simulink library "APST_Lib"  (R2016a)
settings: Solver=ode45  StartTime=0.0  StopTime=10.0  RelTol=1e-3
undefined symbols (not defined in the file or in its folder): ACM, COMP_MAP, rev_comms_sink
libraries: APST_Lib x97
(part 4 of 6)

== system APST_Lib/Thermal Components ==
  "ACM Shaft " : Subsystem  mask(Shaft){N_init=45000, Comp_r1=.05, Comp_r2=.15, m_comp=5, Turb_r1=.15, Turb_r2=.1, m_turb=5, PComp_r1=0.05, PComp_r2=0.025, m_pcomp=5, Shft_r=.05, m_shft=10, J_comp=0.034904, J_turb=0.041645, J_pcomp=0.0041518, J_shaft=0.0125}
      mask prompts: N_init "Initial Rotational Speed [RPM]"; Comp_r1 "Entrance Tip Radius [m]"; Comp_r2 "Exit Tip Radius [m]"; m_comp "Mass [kg]"; Turb_r1 "Entrance Tip Radius [m]"; Turb_r2 "Exit Tip Radius [m]"; m_turb "Mass [kg]"; PComp_r1 "Entrance Tip Radius [m]"; PComp_r2 "Exit Tip Radius [m]"; m_pcomp "Mass [kg]"; Shft_r "Radius [m]"; m_shft "Mass [kg]"; J_comp "Compressor"; J_turb "Expansion Turbine"; J_pcomp "Power Compressor"; J_shaft "ACM Shaft"
      mask init:
      | load Fluids
      | eval(['Air = Fluid.Air;']);
      | 
      | J_comp = (3/10) * m_comp * (Comp_r2^5 - Comp_r1^5) / (Comp_r2^3 - Comp_r1^3);
      | set_param(gcb,'J_comp',num2str(J_comp));
      | 
      | J_turb = (3/10) * m_comp * (Turb_r1^5 - Turb_r2^5) / (Turb_r1^3 - Turb_r2^3);
      | set_param(gcb,'J_turb',num2str(J_turb));
      | 
      | J_pcomp = (3/10) * m_comp * (PComp_r1^5 - PComp_r2^5) / (PComp_r1^3 - PComp_r2^3);
      | set_param(gcb,'J_pcomp',num2str(J_pcomp));
      | 
      | J_shaft = (1/2) * m_shft * Shft_r^2;
      | set_param(gcb,'J_shaft',num2str(J_shaft));
  Air Volume : Subsystem  mask(Air volume){fld=Air, T_init=22, M_init=262.8177, P_init=105, Tamb_init=22, H=0, D=3, L=30, V=212.0575, A_sa=282.7433, Pamb=101, E_fluid=101*1e3}
      mask prompts: fld "Fluid Type"; T_init "Initial Air Temperature [°C]"; M_init "Initial Fluid Mass [kg]"; P_init "Air Pressure [kPa]"; Tamb_init "Initial Ambient Temperature [°C]"; H "Heat Transfer Coefficient with Ambient [W/m²K]"; D "Air Volume Diameter [m]"; L "Air Volume Length [m]"; V "Air Volume [m³]"; A_sa "Air Volume Surface Area [m²]"; Pamb "Ambient Pressure [kPa]"; E_fluid "Bulk Modulus"
      mask help: Tracks the time rate of change for fluid mass and temperature.
      mask init:
      | load('Fluids.mat');
      | Fluid = eval(['Fluid.',fld]);
      | 
      | % calculate the volume -- assuming a cylinder
      | V = L*pi*D^2/4;    
      | set_param(gcb,'V',num2str(V));
      | 
      | % calculate the surface area -- assuming a cylinder
      | SA = L * pi * D ;
      | set_param(gcb,'A_sa',num2str(SA));
      | 
      | % Note: Assumes a fixed initial pressure to calculate density
      | P_for_rho = 105;
      | Rho = qminterp2(Fluid.T, Fluid.P, Fluid.Rho_pt, T_init, P_for_rho);
      | 
      | % set the mass of air in the air volume
      | set_param(gcb,'M_init',num2str(Rho*V));
      settings: OpenFcn=|
      | load('Fluids.mat');
      | Set_Fluid_Popup_Names( Fluid )
      mask TypeOptions fld: Fuel | Water | Air | PG50
      mask DialogControl NomValuesGroupVar Prompt: Component Sizing - Nominal Values
      mask Display:
      | image(imread('cabin.png'))
      | 
      | text(0.5,0.9,['{\bf Air Volume}'],'TexMode','on','horizontalAlignment', 'center')
      | text(0.5,0.1,['{(P)}'],'TexMode','on','horizontalAlignment', 'center')
      | 
      | port_label('input',1,'Flow In')
      | port_label('input',2,'Amb. Temp. [°C]')
      | port_label('input',3,'Q internal [kW]')
      | port_label('output',1,'Flow Out')
      | % port_label('output',2,'Fluid Mass [kg]')
  Cold Plate : Subsystem  mask(Cold Plate){fld=Fuel, P_init=101, Tw_init=22, T_init=22, f=0.05, KL=0, PAF=1, M_wall=0.77632, Cp_wall=.9, H1=2000, D=0.007, L=0.75, t=0.0015, E=2.4e6, v=0.4, dH=0, e_rough=0.0015*1e-3}
      mask prompts: fld "Fluid Type"; P_init "Initial Outlet Pressure [kPa]"; Tw_init "Initial Wall Temperature [°C]"; T_init "Initial Outlet Temperature [°C]"; f "Friction Factor [-]"; KL "Minor Losses [-]"; PAF "HTC Parameter Adjustment Factor [-]"; M_wall "Wall Mass [kg]"; Cp_wall "Wall Specific Heat [kJ/kg*K]"; H1 "Heat Transfer Coeff. [W/m²K]"; D "Internal Diameter [m]"; L "Tube Length [m]"; t "Tube Wall Thickness [m]"; E "Tube Modulus of Elasticity [kPa]"; v "Tube Poisson Ratio [-]"; dH "Height between Inlet and Outlet [m]"; e_rough "Surface Roughness [m] (0.0015mm for copper, 0.01mm for rubber, 0mm for plastic)"
      mask help: Tracks the time rate of change of the pressure, wall temperature, and fluid exit temperature.
      mask init:
      | load('Fluids.mat');
      | Fluid = eval(['Fluid.',fld]);
      | 
      | load('Moody.mat');
      settings: OpenFcn=|
      | load('Fluids.mat');
      | Set_Fluid_Popup_Names( Fluid )
      mask TypeOptions fld: Fuel | Water | Air | PG50
      mask DialogControl Container13 Prompt: Component Sizing - Nominal Values
      mask Display:
      | image(imread('ColdPlate.jpg'))
      | 
      | text(0.5,0.95,['{\bf ',fld,' Cold Plate}'],'TexMode','on','horizontalAlignment', 'center')
      | text(0.5,0.08,['{-----(P)}'],'TexMode','on','horizontalAlignment', 'center')
      | 
      | port_label('input',1,'Flow In')
      | port_label('input',2,'Heat Load [kW]')
      | port_label('output',1,'Flow Out')
  Compressor : Subsystem  mask(Centrifugal Compressor){COMP=ACM.MAP.PwrComp, init_mdot=0}
      mask prompts: COMP "Workspace Variable:"; init_mdot "Initial Mass Flow Rate"
      mask help:
      | Input #1: Flow conditions at compressor inlet [kPa, °C]
      | Input #2: RPM of the compressor shaft [RPM]
      |
      | Output #1: Flow conditions at compressor outlet [kg/s, kPa, °C]
      | Output #2: Power consumed by the compressor [W]
      mask Display:
      | image(imread('compressor.png'))
      | 
      | text(0.5,0.95,['{\bf Compressor}'],'TexMode','on','horizontalAlignment', 'center')
      | text(0.5,0.08,['{----}'],'TexMode','on','horizontalAlignment', 'center')
      | 
      | port_label('input',1,'Flow In')
      | port_label('input',2,'RPM')
      | 
      | port_label('output',1,'Flow Out #')
      | port_label('output',2,'Power [W]')
  Fan : Subsystem  mask(Liquid Pump){P_init=145, T_init=22, D=13*1e-3, L=0.1, rho=1000, cp=4, E=0, Omega_max=3000, DP_max=20, mdot_max=0.5, alpha=0.001}
      mask prompts: P_init "Intial Outlet Pressure [kPa]"; T_init "Intial Outlet Temperature [°C]"; D "Pipe Internal Diameter [m]"; L "Pipe Length [m]"; rho "Air Density [kg/m^3]"; cp "Air Specific Heat [kJ/kgK]"; E "Air Modulus of Elasticity [N/m^2]"; Omega_max "Maximum Shaft Speed [RPM]"; DP_max "Maximum Pressure Difference [kPa]"; mdot_max "Maximum Mass Flow Rate [kg/s]"; alpha "Heat Generation Coefficient [kW/RPM]"
      mask help: Tracks the time rate of change of fluid temperature, mass flow rate, and power consumption.
      mask init:
      | load('Fluids.mat');
      | Fluid = eval(['Fluid.Air']);
      settings: OpenFcn=|
      | load('Fluids.mat');
      | Set_Fluid_Popup_Names( Fluid )
      mask DialogControl Container15 Prompt: Component Sizing - Nominal Values
      mask Display:
      | % image(imread('centpump.jpg'))
      | 
      | text(0.5,0.95,['{\bf Fan}'],'TexMode','on','horizontalAlignment', 'center')
      | text(0.5,0.1,['{-----(P)}'],'TexMode','on','horizontalAlignment', 'center')
      | 
      | port_label('input',1,'Flow In')
      | port_label('input',2,'Power')
      | port_label('input',3,'Shaft Speed [RPM]')
      | port_label('output',1,'Flow Out')
  Flow Split_Junction : Subsystem  mask(Split/Junction){fld=Fuel, Num_Out=1, Num_In=1, P_init=110, T_init=22, D=0.013, L=0.1, t=0.0015, E=2.4e6, v=0.4}
      mask prompts: fld "Fluid Type"; Num_Out "Number of Outlet Flows"; Num_In "Number of Inlet Flows"; P_init "Initial Pressure [kPa]"; T_init "Initial Temperature [°C]"; D "Diameter [m]"; L "Length [m]"; t "Tube Wall Thickness [m]"; E "Tube Modulus of Elasticity [kPa]"; v "Tube Poisson Ratio [-]"
      mask help: Splits and junctions flows using dynamic relationships. Note that the library link of the block is disabled when it is imported into a model.
      mask init:
      | h      = get_param(gcb,'handle');   % Get block handle
      | blk    = gcb;
      | hblock = get(h);     % Parse out handles structure
      | 
      | load('Fluids.mat');
      | Fluid = eval(['Fluid.',fld]);
      | 
      | % delete any previous inports and bus selectors
      | for i = str2num(hblock.Num_In)+1:hblock.Ports(1)
      |     delete_block([blk,'/In',num2str(i)])
      |     delete_block([blk,'/gb',num2str(i)])
      |     delete_block([blk,'/gm',num2str(i)])
      |     delete_block([blk,'/gt',num2str(i)])
      |     delete_block([blk,'/gp',num2str(i)])
      |     delete_block([blk,'/Sink',num2str(i)])
      |     delete_block([blk,'/pout',num2str(i)])
      |     delete_block([blk,'/min',num2str(i)])
      |     delete_block([blk,'/tin',num2str(i)])
      |     
      |     delete_unconnected_lines(blk)
      | end
      | 
      | % delete any previous inports and bus selectors
      | for i = str2num(hblock.Num_Out)+1:hblock.Ports(2)
      |     delete_block([blk,'/Out',num2str(i)])
      |     delete_block([blk,'/m',num2str(i)])
      |     delete_block([blk,'/t',num2str(i)])
      |     delete_block([blk,'/p',num2str(i)])
      |     delete_block([blk,'/b',num2str(i)])
      |     delete_block([blk,'/Source',num2str(i)])
      |     delete_block([blk,'/g',num2str(i)])
      |     delete_block([blk,'/mout',num2str(i)])
      |     %delete_block([blk,'/tout',num2str(i)])
      |     
      |     delete_unconnected_lines(blk)
      | end
      | 
      | set_param([blk,'/Mux_In_1'],'Inputs',hblock.Num_In)
      | set_param([blk,'/Mux_In_2'],'Inputs',hblock.Num_Out)
      | set_param([blk,'/Mux_In_3'],'Inputs',hblock.Num_In)
      | %set_param([blk,'/Mux_Out_1'],'Outputs',hblock.Num_Out)
      | 
      | % generate inports, bus selectors, and route lines to each vector concat
      | for i = hblock.Ports(1)+1:str2num(hblock.Num_In)
      |     
      |     % add blocks
      |     add_block('simulink/Ports & Subsystems/In1',   [blk,'/In',num2str(i)],    'Position',[120 i*80-25+20 150 i*80-12+20]);         % adding inport
      |     add_block([blk,'/gb1'],                        [blk,'/gb',num2str(i)],   'Position',[200 i*80-20+20-18 205 i*80-2+20+2]);         % adding inport
      |     add_block('simulink/Signal Routing/Goto',      [blk,'/gm',num2str(i)],    'Position',[260 i*80-17 340 i*80-3]);         % adding inport
      |     add_block('simulink/Signal Routing/Goto',      [blk,'/gt',num2str(i)],    'Position',[260 i*80+3 340 i*80+17]);         % adding inport
      |     add_block('simulink/Sinks/Terminator',          [blk,'/gp',num2str(i)],    'Position',[260 i*80+23 280 i*80+37]);         % adding inport
      |     add_block('APST_Lib/Support Components/Sink',[blk,'/Sink',num2str(i)],'Position',[745 i*80-14 810 i*80+14]);         % adding inport
      |     add_block('simulink/Signal Routing/From',      [blk,'/pout',num2str(i)],    'Position',[625 i*80-14 705 i*80+14]);         % adding inport
      |     add_block('simulink/Signal Routing/From',       [blk,'/min',num2str(i)],     'Position',[935 -258+i*20 1015 -242+i*20]);         % adding inport
      |     add_block('simulink/Signal Routing/From',       [blk,'/tin',num2str(i)],     'Position',[935 1+i*20 1015 19+i*20]);         % adding inport
      |     
      |     % set goto and from tags
      |     set_param([blk,'/gm',num2str(i)],'GotoTag',char(horzcat('M_in',num2str(i))))
      |     set_param([blk,'/gt',num2str(i)],'GotoTag',char(horzcat('T_in',num2str(i))))
      |     %set_param([blk,'/gp',num2str(i)],'GotoTag',char(horzcat('P_in',num2str(i))))
      |     set_param([blk,'/pout',num2str(i)],'GotoTag',char('P'))
      |     set_param([blk,'/min',num2str(i)],'GotoTag',char(horzcat('M_in',num2str(i))))
      |     set_param([blk,'/tin',num2str(i)],'GotoTag',char(horzcat('T_in',num2str(i))))
      |     
      |     % set goto and from background colors
      |     set_param([blk,'/gm',num2str(i)],'BackgroundColor','yellow')
      |     set_param([blk,'/gt',num2str(i)],'BackgroundColor','yellow')
      |     %set_param([blk,'/gp',num2str(i)],'BackgroundColor','yellow')
      |     set_param([blk,'/min',num2str(i)],'BackgroundColor','yellow')
      |     set_param([blk,'/tin',num2str(i)],'BackgroundColor','yellow')
      |     set_param([blk,'/pout',num2str(i)],'BackgroundColor','cyan')
      |     
      |     % add lines
      |     add_line(blk,['In',num2str(i),'/1'], ['gb',num2str(i),'/1'],'AutoRouting','on')
      |     add_line(blk,['gb',num2str(i),'/1'],  ['gm',num2str(i),'/1'],'AutoRouting','on')
      |     add_line(blk,['gb',num2str(i),'/2'],  ['gt',num2str(i),'/1'],'AutoRouting','on')
      |     add_line(blk,['gb',num2str(i),'/3'],  ['gp',num2str(i),'/1'],'AutoRouting','on')
      |     add_line(blk,['pout',num2str(i),'/1'],  ['Sink',num2str(i),'/1'],'AutoRouting','on')
      |     add_line(blk,['min',num2str(i),'/1'],  ['Mux_In_1/',num2str(i)],'AutoRouting','on')
      |     add_line(blk,['tin',num2str(i),'/1'],  ['Mux_In_3/',num2str(i)],'AutoRouting','on')
      |     
      | end
      | 
      | % generate inports, bus selectors, and route lines to each vector concat
      | for i = hblock.Ports(2)+1:str2num(hblock.Num_Out)
      |     
      |     % add blocks
      |     add_block('simulink/Ports & Subsystems/Out1',   [blk,'/Out',num2str(i)],   'Position',[30 i*80-25+20 60 i*80-12+20]);         % adding inport
      |     add_block('simulink/Signal Routing/From',       [blk,'/m',num2str(i)],     'Position',[-150 i*80-20 -70 i*80-2]);         % adding inport
      |     add_block('simulink/Signal Routing/From',       [blk,'/t',num2str(i)],     'Position',[-150 i*80-20+20 -70 i*80-2+20]);         % adding inport
      |     add_block('simulink/Signal Routing/From',       [blk,'/p',num2str(i)],     'Position',[-150 i*80-20+40 -70 i*80-2+40]);         % adding inport
      |     add_block('simulink/Signal Routing/Bus Creator',[blk,'/b',num2str(i)],     'Position',[5 i*80-20+20-18 10 i*80-2+20+2]);         % adding inport
      |     add_block('APST_Lib/Support Components/Source',[blk,'/Source',num2str(i)],'Position',[395 i*80-14 460 i*80+14]);         % adding inport
      |     add_block('simulink/Signal Routing/Goto',       [blk,'/g',num2str(i)],     'Position',[505 i*80-9 585 i*80+9]);         % adding inport
      |     add_block('simulink/Signal Routing/From',       [blk,'/mout',num2str(i)],  'Position',[935 -129+i*20 1015 -111+i*20]);         % adding inport
      |     %add_block('simulink/Signal Routing/Goto',      [blk,'/tout',num2str(i)],   'Position',[1455 -259+i*20 1535 -241+i*20]);         % adding inport
      |     
      |     % set goto and from tags
      |     set_param([blk,'/m',num2str(i)],'GotoTag',char(horzcat('M_out',num2str(i))))
      |     %set_param([blk,'/t',num2str(i)],'GotoTag',char(horzcat('T_out',num2str(i))))
      |     set_param([blk,'/t',num2str(i)],'GotoTag',char('T'))
      |     set_param([blk,'/p',num2str(i)],'GotoTag',char('P'))
      |     set_param([blk,'/g',num2str(i)],'GotoTag',char(horzcat('M_out',num2str(i))))
      |     set_param([blk,'/mout',num2str(i)],'GotoTag',char(horzcat('M_out',num2str(i))))
      |     %set_param([blk,'/tout',num2str(i)],'GotoTag',char(horzcat('T_out',num2str(i))))
      |     set_param([blk,'/b',num2str(i)],'Inputs','3')
      |     
      |     % set goto and from background colors
      |     set_param([blk,'/t',num2str(i)],'BackgroundColor','cyan')
      |     set_param([blk,'/m',num2str(i)],'BackgroundColor','cyan')
      |     set_param([blk,'/p',num2str(i)],'BackgroundColor','cyan')
      |     set_param([blk,'/g',num2str(i)],'BackgroundColor','cyan')
      |     set_param([blk,'/mout',num2str(i)],'BackgroundColor','cyan')
      |     %set_param([blk,'/tout',num2str(i)],'BackgroundColor','cyan')
      |     
      |     % add lines
      |     add_line(blk,['m',num2str(i),'/1'],['b',num2str(i),'/1'],'AutoRouting','on')
      |     p = get_param([blk,'/m',num2str(i)],'PortHandles');
      |     l = get_param(p.Outport,'Line');
      |     set_param(l,'Name','mdot_kgps')
      |     
      |     add_line(blk,['t',num2str(i),'/1'],['b',num2str(i),'/2'],'AutoRouting','on')
      |     p = get_param([blk,'/t',num2str(i)],'PortHandles');
      |     l = get_param(p.Outport,'Line');
      |     set_param(l,'Name','T_C')
      |     
      |     add_line(blk,['p',num2str(i),'/1'],['b',num2str(i),'/3'],'AutoRouting','on')
      |     p = get_param([blk,'/p',num2str(i)],'PortHandles');
      |     l = get_param(p.Outport,'Line');
      |     set_param(l,'Name','P_kPa')
      |     
      |     add_line(blk,['b',num2str(i),'/1'],['Out',num2str(i),'/1'],'AutoRouting','on')
      |     add_line(blk,['Source',num2str(i),'/1'],['g',num2str(i),'/1'],'AutoRouting','on')
      |     add_line(blk,['mout',num2str(i),'/1'],  ['Mux_In_2/',num2str(i)],'AutoRouting','on')
      |     %add_line(blk,['Mux_Out_1/',num2str(i)], ['tout',num2str(i),'/1'],'AutoRouting','on')
      | end
      | 
      | try
      |     set_param([blk,'/Selector1'],'InputPortWidth',num2str(hblock.Num_In))
      |     set_param([blk,'/Selector2'],'InputPortWidth',num2str(hblock.Num_In))
      |     
      |     selector_str = '[1 ';
      |     for i = 2:str2num(hblock.Num_In)
      |         selector_str = [selector_str,num2str(i),' '];
      |     end
      |     selector_str = [selector_str,']'];
      |     set_param([blk,'/Selector1'],'IndexParamArray',{selector_str})%num2cell(1:hblock.Num_In))
      |     set_param([blk,'/Selector2'],'IndexParamArray',{selector_str})%num2cell(1:hblock.Num_In))
      | catch
      |     selector_str = '[1 ';
      |     for i = 2:str2num(hblock.Num_In)
      |         selector_str = [selector_str,num2str(i),' '];
      |     end
      |     selector_str = [selector_str,']'];
      |     set_param([blk,'/Selector1'],'IndexParamArray',{selector_str})%num2cell(1:hblock.Num_In))
      |     set_param([blk,'/Selector2'],'IndexParamArray',{selector_str})%num2cell(1:hblock.Num_In))
      |     
      |     set_param([blk,'/Selector1'],'InputPortWidth',num2str(hblock.Num_In))
      |     set_param([blk,'/Selector2'],'InputPortWidth',num2str(hblock.Num_In))
      | end 
      |     
      |     clear h blk hblock
      settings: CopyFcn=|
      | h      = get_param(gcb,'handle');   % Get block handle
      | blk    = gcb;
      | 
      | set_param(blk, 'LinkStatus', 'inactive')
      settings: OpenFcn=|
      | load('Fluids.mat');
      | Set_Fluid_Popup_Names( Fluid )
      mask TypeOptions fld: Fuel | Water | Air | PG50
      mask DialogControl Container15 Prompt: Component Sizing - Nominal Values
      mask Display:
      | image(imread('Split.jpg'));
      | 
      | text(0.5,0.95,['{\bf',fld,' Split/Junction}'],'TexMode','on','horizontalAlignment', 'center')
      | text(0.5,0.08,['{(P)}'],'TexMode','on','horizontalAlignment', 'center')
      | 
      | h      = get_param(gcb,'handle');   % Get block handle
      | blk    = gcb;
      | hblock = get(h);     % Parse out handles structure
      | for i = 1:str2num(hblock.Num_In)
      |     port_label('input',i,horzcat('Flow In #',num2str(i)))
      | end
      | for i = 1:str2num(hblock.Num_Out)
      |     port_label('output',i,horzcat('Flow Out #',num2str(i)))
      | end
  Flow Split_Junction1 : Subsystem  mask(Split/Junction){fld=Fuel, Num_Out=2, Num_In=1, P_init=110, T_init=22, D=0.013, L=0.1, t=0.0015, E=2.4e6, v=0.4}
      mask prompts: fld "Fluid Type"; Num_Out "Number of Outlet Flows"; Num_In "Number of Inlet Flows"; P_init "Initial Pressure [kPa]"; T_init "Initial Temperature [°C]"; D "Diameter [m]"; L "Length [m]"; t "Tube Wall Thickness [m]"; E "Tube Modulus of Elasticity [kPa]"; v "Tube Poisson Ratio [-]"
      mask help: Splits and junctions flows using dynamic relationships. Note that the library link of the block is disabled when it is imported into a model.
      mask init:
      | h      = get_param(gcb,'handle');   % Get block handle
      | blk    = gcb;
      | hblock = get(h);     % Parse out handles structure
      | 
      | load('Fluids.mat');
      | Fluid = eval(['Fluid.',fld]);
      | 
      |     
      |     clear h blk hblock
      settings: CopyFcn=|
      | h      = get_param(gcb,'handle');   % Get block handle
      | blk    = gcb;
      | 
      | set_param(blk, 'LinkStatus', 'inactive')
      settings: OpenFcn=|
      | load('Fluids.mat');
      | Set_Fluid_Popup_Names( Fluid )
      mask TypeOptions fld: Fuel | Water | Air | PG50
      mask DialogControl Container15 Prompt: Component Sizing - Nominal Values
      mask Display:
      | image(imread('valve.png'));
      | 
      | text(0.5,0.95,['{\bf',fld,' Valve}'],'TexMode','on','horizontalAlignment', 'center')
      | text(0.5,0.08,['{----}'],'TexMode','on','horizontalAlignment', 'center')
      | 
      | h      = get_param(gcb,'handle');   % Get block handle
      | blk    = gcb;
      | hblock = get(h);     % Parse out handles structure
      | for i = 1:str2num(hblock.Num_In)
      |     port_label('input',i,horzcat('Flow In #',num2str(i)))
      | end
      | port_label('input',2,'Input [0-1]')
      | for i = 1:str2num(hblock.Num_Out)
      |     port_label('output',i,horzcat('Flow Out #',num2str(i)))
      | end
  Fluid Tank : Subsystem  mask(Fluid Tank){fld=Fuel, T_init=22, h_init=0.2, M_init=500, P_init=105, Tamb_init=22, H=0, D=0.08, V=3, A_sa=0, Pamb=101}
      mask prompts: fld "Fluid Type"; T_init "Initial Fluid Temperature [°C]"; h_init "Initial Fluid Height [m]"; M_init "Initial Fluid Mass [kg]"; P_init "Tank Pressure [kPa]"; Tamb_init "Initial Ambient Temperature [°C]"; H "Heat Transfer Coefficient with Ambient [W/m²K]"; D "Tank Diameter [m]"; V "Tank Volume [m³]"; A_sa "Tank Surface Area [m²]"; Pamb "Ambient Pressure [kPa]"
      mask help: Tracks the time rate of change for fluid mass and temperature.
      mask init:
      | load('Fluids.mat');
      | Fluid = eval(['Fluid.',fld]);
      | 
      | % Note: Assumes a fixed initial pressure to calculate density
      | P_for_rho = 105;
      | Rho = qminterp2(Fluid.T, Fluid.P, Fluid.Rho_pt, T_init, P_for_rho);
      | 
      | % M_init = h_init*Rho*pi*D^2/4;
      | M_max = Rho*V;
      | if M_max < M_init
      |     set_param(gcb,'M_init',num2str(M_max));
      |     msgbox('Fuel tank volume is too small for initial mass. Setting initial mass to maximum.')
      | end
      | 
      | % P_init = Rho*9.81*h_init/1000 + Pamb;
      | % set_param(gcb,'P_init',num2str(P_init));
      settings: OpenFcn=|
      | load('Fluids.mat');
      | Set_Fluid_Popup_Names( Fluid )
      mask TypeOptions fld: Fuel | Water | Air | PG50
      mask DialogControl NomValuesGroupVar Prompt: Component Sizing - Nominal Values
      mask Display:
      | image(imread('fueltank.jpg'))
      | 
      | text(0.5,0.9,['{\bf ',fld,' Tank}'],'TexMode','on','horizontalAlignment', 'center')
      | text(0.5,0.1,['{(P)}'],'TexMode','on','horizontalAlignment', 'center')
      | 
      | port_label('input',1,'Flow In')
      | port_label('input',2,'Amb. Temp. [°C]')
      | port_label('input',3,'Q internal [kW]')
      | port_label('output',1,'Flow Out')
      | port_label('output',2,'Fluid Mass [kg]')
  Heat Exchanger : Subsystem  mask(Heat Exchanger){Tw_init=22, fld1=Air, P1_init=95, T1_init=22, f1=0.05, KL1=0, fld2=Air, P2_init=120, T2_init=10, f2=0.05, KL2=0, M_wall=0.1, Cp_wall=0.9, Pass1=5, H1=2000, b1=1*1e-3, W1=87*1e-3, L1=0.193, dH1=0, e1=0.0015*1e-3, Nu_lam1=5.6153, Pass2=5, H2=2000, b2=1*1e-2, W2=87*1e-2, L2=0.193, dH2=0, e2=0.0015*1e-3, Nu_lam2=5.6153}
      mask prompts: Tw_init "Initial Wall Temperature [°C]"; fld1 "Fluid Type 1"; P1_init "Initial Outlet 1 Pressure [kPa]"; T1_init "Initial Outlet 1 Temperature [°C]"; f1 "Friction Factor [-]"; KL1 "Minor Losses [-]"; fld2 "Fluid Type 2"; P2_init "Initial Outlet 2 Pressure [kPa]"; T2_init "Initial Outlet 2 Temperature [°C]"; f2 "Friction Factor [-]"; KL2 "Minor Losses [-]"; M_wall "Single Wall Mass [kg]"; Cp_wall "Wall Specific Heat [kJ/kg*K]"; Pass1 "Number of Passes"; H1 "Heat transfer coeff. [W/m²K]"; b1 "Plate Spacing [m]"; W1 "Plate Width [m]"; L1 "Plate Length [m]"; dH1 "Height between Inlet and Outlet [m]"; e1 "Surface Roughness [m] (0.0015mm for copper, 0.01mm for rubber, 0mm for plastic)"; Nu_lam1 "Laminar Nu"; Pass2 "Number of Passes"; H2 "Heat transfer coeff. [W/m²K]"; b2 "Plate Spacing [m]"; W2 "Plate Width [m]"; L2 "Plate Length [m]"; dH2 "Height between Inlet and Outlet [m]"; e2 "Surface Roughness [m] (0.0015mm for copper, 0.01mm for rubber, 0mm for plastic)"; Nu_lam2 "Laminar Nu"
      mask help: Tracks the time rate of change of the pressure, wall temperature, and exit flow temperatures.
      mask init:
      | load('Fluids.mat');
      | Fluid1 = eval(['Fluid.',fld1]);
      | Fluid2 = eval(['Fluid.',fld2]);
      | 
      | load('Moody.mat');
      | 
      | load('Laminar_Props.mat')
      | Nu_lam1 = interp1(LamProps.b_a,LamProps.Nu,max(W1,b1)/min(W1,b1));
      | Nu_lam2 = interp1(LamProps.b_a,LamProps.Nu,max(W2,b2)/min(W2,b2));
      | set_param(gcb,'Nu_lam1',num2str(Nu_lam1));
      | set_param(gcb,'Nu_lam2',num2str(Nu_lam2));
      settings: OpenFcn=|
      | load('Fluids.mat');
      | Set_Fluid_Popup_Names( Fluid )
      mask TypeOptions fld1: Fuel | Water | Air | PG50
      mask TypeOptions fld2: Fuel | Water | Air | PG50
      mask DialogControl Container18 Prompt: Side 1
      mask DialogControl Container17 Prompt: Side 2
      mask DialogControl Container14 Prompt: Component Sizing - Nominal Values
      mask DialogControl Container8 Prompt: Side 1
      mask DialogControl Container9 Prompt: Side 2
      mask Display:
      | image(imread('HX.jpg'))
      | 
      | text(0.5,0.95,['{\bf ',fld1,'/',fld2,' HX}'],'TexMode','on','horizontalAlignment', 'center')
      | text(0.5,0.08,['{-----(P)}'],'TexMode','on','horizontalAlignment', 'center')
      | 
      | port_label('input',1,['In 1 (',fld1,')'])
      | port_label('input',2,['In 2 (',fld2,')'])
      | port_label('output',1,['Out 1 (',fld1,')'])
      | port_label('output',2,['Out 2 (',fld2,')'])
  Pipe_P_to_M : Subsystem  mask(Pipe (P to M)){fld=Fuel, T_init=22, P_init=101, Tamb_init=22, f=0.05, KL_tube=0, KL=0, H=0, D=13*1e-3, L=0.1, t=0.0015, E=2.4e6, v=0.4, dH=0, e_rough=0.01*1e-3, Num_MFRS=0, Num_PS=0, Num_TS=0, Num_BV=0, Num_CV=0}
      mask prompts: fld "Fluid Type"; T_init "Initial Outlet Temperature [°C]"; P_init "Initial Outlet Pressure [kPa]"; Tamb_init "Initial Ambient Temperature [°C]"; f "Tube Friction Factor [-]"; KL_tube "Tube Minor Losses [-]"; KL "Total Minor Losses [-]"; H "Heat Transfer Coefficient [W/m²K]"; D "Pipe Internal Diameter [m]"; L "Pipe Length [m]"; t "Tube Wall Thickness [m]"; E "Tube Modulus of Elasticity [kPa]"; v "Tube Poisson Ratio [-]"; dH "Height between Inlet and Outlet [m]"; e_rough "Surface Roughness [m] (0.0015mm for copper, 0.01mm for rubber, 0mm for plastic)"; Num_MFRS "Number of Mass Flow Rate Sensors"; Num_PS "Number of Pressure Sensors"; Num_TS "Number of Temperature Sensors"; Num_BV "Number of Ball Valves"; Num_CV "Number of Check Valves"
      mask help: Models a pipe given an upstream pressure and downstream mass flow rate.
      mask init:
      | load('Fluids.mat');
      | Fluid = eval(['Fluid.',fld]);
      | 
      | load('Moody.mat');
      | 
      | KL = KL_correction(KL_tube,Num_MFRS,Num_PS,Num_TS,Num_BV,Num_CV);
      | set_param(gcb,'KL',num2str(KL));
      settings: OpenFcn=|
      | load('Fluids.mat');
      | Set_Fluid_Popup_Names( Fluid )
      mask TypeOptions fld: Fuel | Water | Air | PG50
      mask DialogControl NomValuesGroupVar Prompt: Component Sizing - Nominal Values
      mask Display:
      | if sum([Num_MFRS,Num_PS,Num_TS,Num_BV,Num_CV])==0
      |     image(imread('Tube.jpg'))
      | elseif sum([Num_MFRS,Num_PS,Num_TS])~=0 && sum([Num_BV,Num_CV])==0
      |     image(imread('Tube_Sensor.jpg'))
      | elseif sum([Num_MFRS,Num_PS,Num_TS])==0 && sum([Num_BV,Num_CV])~=0
      |     image(imread('Tube_Valve.jpg'))
      | else
      |     image(imread('Tube_Valve_Sensor.jpg'))
      | end
      | 
      | text(0.5,0.95,['{\bf ',fld,' Pipe (P to M)}'],'TexMode','on','horizontalAlignment', 'center')
      | text(0.5,0.1,['{-----(P)}'],'TexMode','on','horizontalAlignment', 'center')
      | 
      | port_label('input',1,'Flow In')
      | % port_label('input',2,'Amb. Temp. [°C]')
      | port_label('output',1,'Flow Out')
  Pipe_P_to_P : Subsystem  mask(Pipe (P to P)){fld=Fuel, T_init=22, Tamb_init=22, f=0.05, KL_tube=0, KL=0, H=0, D=13*1e-3, L=0.1, t=0.0015, E=2.4e6, v=0.4, dH=0, e_rough=0.01*1e-3, Num_MFRS=0, Num_PS=0, Num_TS=0, Num_BV=0, Num_CV=0}
      mask prompts: fld "Fluid Type"; T_init "Initial Outlet Temperature [°C]"; Tamb_init "Initial Ambient Temperature [°C]"; f "Tube Friction Factor [-]"; KL_tube "Tube Minor Losses [-]"; KL "Total Minor Losses [-]"; H "Heat Transfer Coefficient [W/m²K]"; D "Pipe Internal Diameter [m]"; L "Pipe Length [m]"; t "Tube Wall Thickness [m]"; E "Tube Modulus of Elasticity [kPa]"; v "Tube Poisson Ratio [-]"; dH "Height between Inlet and Outlet [m]"; e_rough "Surface Roughness [m] (0.0015mm for copper, 0.01mm for rubber, 0mm for plastic)"; Num_MFRS "Number of Mass Flow Rate Sensors"; Num_PS "Number of Pressure Sensors"; Num_TS "Number of Temperature Sensors"; Num_BV "Number of Ball Valves"; Num_CV "Number of Check Valves"
      mask help: Models a pipe given upstream and downstream pressures.
      mask init:
      | load('Fluids.mat');
      | Fluid = eval(['Fluid.',fld]);
      | 
      | load('Moody.mat');
      | 
      | KL = KL_correction(KL_tube,Num_MFRS,Num_PS,Num_TS,Num_BV,Num_CV);
      | set_param(gcb,'KL',num2str(KL));
      settings: OpenFcn=|
      | load('Fluids.mat');
      | Set_Fluid_Popup_Names( Fluid )
      mask TypeOptions fld: Fuel | Water | Air | PG50
      mask DialogControl NomValuesGroupVar Prompt: Component Sizing - Nominal Values
      mask Display:
      | if sum([Num_MFRS,Num_PS,Num_TS,Num_BV,Num_CV])==0
      |     image(imread('Tube.jpg'))
      | elseif sum([Num_MFRS,Num_PS,Num_TS])~=0 && sum([Num_BV,Num_CV])==0
      |     image(imread('Tube_Sensor.jpg'))
      | elseif sum([Num_MFRS,Num_PS,Num_TS])==0 && sum([Num_BV,Num_CV])~=0
      |     image(imread('Tube_Valve.jpg'))
      | else
      |     image(imread('Tube_Valve_Sensor.jpg'))
      | end
      | 
      | text(0.5,0.95,['{\bf ',fld,' Pipe (P to P)}'],'TexMode','on','horizontalAlignment', 'center')
      | text(0.5,0.1,['{-----}'],'TexMode','on','horizontalAlignment', 'center')
      | 
      | port_label('input',1,'Flow In')
      | % port_label('input',2,'Amb. Temp. [°C]')
      | port_label('output',1,'Flow Out')
  Pump1 : Subsystem  mask(Liquid Pump){fld=Fuel, P_init=145, T_init=22, D=13*1e-3, L=0.1, rho=1000, cp=4, E=0, Omega_max=3000, DP_max=20, mdot_max=0.5, alpha=0.001}
      mask prompts: fld "Fluid Type"; P_init "Intial Outlet Pressure [kPa]"; T_init "Intial Outlet Temperature [°C]"; D "Pipe Internal Diameter [m]"; L "Pipe Length [m]"; rho "Fluid Density [kg/m^3]"; cp "Fluid Specific Heat [kJ/kgK]"; E "Fluid Modulus of Elasticity [N/m^2]"; Omega_max "Maximum Shaft Speed [RPM]"; DP_max "Maximum Pressure Difference [kPa]"; mdot_max "Maximum Mass Flow Rate [kg/s]"; alpha "Heat Generation Coefficient [kW/RPM]"
      mask help: Tracks the time rate of change of fluid temperature, mass flow rate, and power consumption.
      mask init:
      | load('Fluids.mat');
      | Fluid = eval(['Fluid.',fld]);
      settings: OpenFcn=|
      | load('Fluids.mat');
      | Set_Fluid_Popup_Names( Fluid )
      mask TypeOptions fld: Fuel | Water | Air | PG50
      mask DialogControl Container15 Prompt: Component Sizing - Nominal Values
      mask Display:
      | image(imread('centpump.jpg'))
      | 
      | text(0.5,0.95,['{\bf ',fld,' Pump}'],'TexMode','on','horizontalAlignment', 'center')
      | text(0.5,0.1,['{-----(P)}'],'TexMode','on','horizontalAlignment', 'center')
      | 
      | port_label('input',1,'Flow In')
      | port_label('input',2,'Power')
      | port_label('input',3,'Shaft Speed [RPM]')
      | port_label('output',1,'Flow Out')
  Turbine : Subsystem  mask(Centrifual Turbine){TURB=ACM.MAP.Turb}
      mask prompts: TURB "Workspace Variable:"
      mask help:
      | Input #1: Flow conditions at turbine inlet [kPa, °C]
      | Input #2: RPM of the turbine shaft [RPM]
      |
      | Output #1: Flow conditions at turbine outlet [kg/s, kPa, °C]
      | Output #2: Power produced by the turbine [W]
      mask Display:
      | image(imread('turbine.png'))
      | 
      | text(0.5,0.95,['{\bf Turbine}'],'TexMode','on','horizontalAlignment', 'center')
      | text(0.5,0.08,['{----}'],'TexMode','on','horizontalAlignment', 'center')
      | 
      | port_label('input',1,'Flow In')
      | port_label('input',2,'RPM')
      | 
      | port_label('output',1,'Flow Out')
      | port_label('output',2,'Power [W]')
  Valve : Subsystem  mask(Solenoid Valve (P to P)){fld=Fuel, T_init=22, f=0.05, KL=0, D=0.013, L=0.1}
      mask prompts: fld "Fluid Type"; T_init "Initial Outlet Temperature [°C]"; f "Friction Factor [-]"; KL "Minor Losses [-]"; D "Internal Diameter [m]"; L "Length [m]"
      mask help: Models an on/off solenoid valve given upstream and downstream pressures.
      mask init:
      | load('Fluids.mat');
      | Fluid = eval(['Fluid.',fld]);
      | 
      | load('Moody.mat');
      settings: OpenFcn=|
      | load('Fluids.mat');
      | Set_Fluid_Popup_Names( Fluid )
      mask TypeOptions fld: Fuel | Water | Air | PG50
      mask DialogControl NomValuesGroupVar Prompt: Component Sizing - Nominal Values
      mask Display:
      | image(imread('Solenoid.jpg'))
      | 
      | 
      | text(0.5,0.95,['{\bf ',fld,' Pipe (P to P)}'],'TexMode','on','horizontalAlignment', 'center')
      | text(0.5,0.1,['{-----}'],'TexMode','on','horizontalAlignment', 'center')
      | 
      | port_label('input',1,'Flow In')
      | port_label('input',2,'Off/On [0,1]')
      | port_label('output',1,'Flow Out')
  Valve1 : Subsystem  mask(Split/Junction){fld=Fuel, Num_Out=1, Num_In=2, P_init=100, T_init=22, D=0.05, L=0.1, t=0.0015, E=2.4e6, v=0.4}
      mask prompts: fld "Fluid Type"; Num_Out "Number of Outlet Flows"; Num_In "Number of Inlet Flows"; P_init "Initial Pressure [kPa]"; T_init "Initial Temperature [°C]"; D "Diameter [m]"; L "Length [m]"; t "Tube Wall Thickness [m]"; E "Tube Modulus of Elasticity [kPa]"; v "Tube Poisson Ratio [-]"
      mask help: Splits and junctions flows using dynamic relationships. Note that the library link of the block is disabled when it is imported into a model.
      mask init:
      | h      = get_param(gcb,'handle');   % Get block handle
      | blk    = gcb;
      | hblock = get(h);     % Parse out handles structure
      | 
      | load('Fluids.mat');
      | Fluid = eval(['Fluid.',fld]);
      | 
      |     
      |     clear h blk hblock
      settings: CopyFcn=|
      | h      = get_param(gcb,'handle');   % Get block handle
      | blk    = gcb;
      | 
      | set_param(blk, 'LinkStatus', 'inactive')
      settings: OpenFcn=|
      | load('Fluids.mat');
      | Set_Fluid_Popup_Names( Fluid )
      mask TypeOptions fld: Fuel | Water | Air | PG50
      mask DialogControl Container15 Prompt: Component Sizing - Nominal Values
      mask Display:
      | image(imread('valve.png'));
      | 
      | text(0.5,0.95,['{\bf',fld,' Valve}'],'TexMode','on','horizontalAlignment', 'center')
      | text(0.5,0.08,['{----(P)}'],'TexMode','on','horizontalAlignment', 'center')
      | 
      | h      = get_param(gcb,'handle');   % Get block handle
      | blk    = gcb;
      | hblock = get(h);     % Parse out handles structure
      | for i = 1:str2num(hblock.Num_In)
      |     port_label('input',i,horzcat('Flow In #',num2str(i)))
      | end
      | port_label('input',3,'Input [0-1]')
      | for i = 1:str2num(hblock.Num_Out)
      |     port_label('output',i,'Flow Out')
      | end
  Valve2 : Subsystem  mask(Split/Junction){fld=Fuel, Num_Out=1, Num_In=1, P_init=100, T_init=22, D=0.05, L=0.1, t=0.0015, E=2.4e6, v=0.4}
      mask prompts: fld "Fluid Type"; Num_Out "Number of Outlet Flows"; Num_In "Number of Inlet Flows"; P_init "Initial Pressure [kPa]"; T_init "Initial Temperature [°C]"; D "Diameter [m]"; L "Length [m]"; t "Tube Wall Thickness [m]"; E "Tube Modulus of Elasticity [kPa]"; v "Tube Poisson Ratio [-]"
      mask help: Splits and junctions flows using dynamic relationships. Note that the library link of the block is disabled when it is imported into a model.
      mask init:
      | h      = get_param(gcb,'handle');   % Get block handle
      | blk    = gcb;
      | hblock = get(h);     % Parse out handles structure
      | 
      | load('Fluids.mat');
      | Fluid = eval(['Fluid.',fld]);
      | 
      |     
      |     clear h blk hblock
      settings: CopyFcn=|
      | h      = get_param(gcb,'handle');   % Get block handle
      | blk    = gcb;
      | 
      | set_param(blk, 'LinkStatus', 'inactive')
      settings: OpenFcn=|
      | load('Fluids.mat');
      | Set_Fluid_Popup_Names( Fluid )
      mask TypeOptions fld: Fuel | Water | Air | PG50
      mask DialogControl Container15 Prompt: Component Sizing - Nominal Values
      mask Display:
      | image(imread('valve.png'));
      | 
      | text(0.5,0.95,['{\bf',fld,' Valve}'],'TexMode','on','horizontalAlignment', 'center')
      | text(0.5,0.08,['{----(P)}'],'TexMode','on','horizontalAlignment', 'center')
      | 
      | h      = get_param(gcb,'handle');   % Get block handle
      | blk    = gcb;
      | hblock = get(h);     % Parse out handles structure
      | for i = 1:str2num(hblock.Num_In)
      |     port_label('input',i,horzcat('Flow In #',num2str(i)))
      | end
      | port_label('input',2,'Input [0-1]')
      | for i = 1:str2num(hblock.Num_Out)
      |     port_label('output',i,'Flow Out')
      | end
  Valve3 : Subsystem  mask(Valve 3in/1out){fld=Fuel, Num_Out=1, Num_In=3, P_init=100, T_init=22, D=0.05, L=0.1, t=0.0015, E=2.4e6, v=0.4}
      mask prompts: fld "Fluid Type"; Num_Out "Number of Outlet Flows"; Num_In "Number of Inlet Flows"; P_init "Initial Pressure [kPa]"; T_init "Initial Temperature [°C]"; D "Diameter [m]"; L "Length [m]"; t "Tube Wall Thickness [m]"; E "Tube Modulus of Elasticity [kPa]"; v "Tube Poisson Ratio [-]"
      mask help: Input should sum to 1. Input is the ratio of flow from each source.
      mask init:
      | h      = get_param(gcb,'handle');   % Get block handle
      | blk    = gcb;
      | hblock = get(h);     % Parse out handles structure
      | 
      | load('Fluids.mat');
      | Fluid = eval(['Fluid.',fld]);
      | 
      |     
      |     clear h blk hblock
      settings: CopyFcn=|
      | h      = get_param(gcb,'handle');   % Get block handle
      | blk    = gcb;
      | 
      | % set_param(blk, 'LinkStatus', 'inactive')
      settings: OpenFcn=|
      | load('Fluids.mat');
      | Set_Fluid_Popup_Names( Fluid )
      mask TypeOptions fld: Fuel | Water | Air | PG50
      mask DialogControl Container15 Prompt: Component Sizing - Nominal Values
      mask Display:
      | image(imread('valve.png'));
      | 
      | text(0.5,0.95,['{\bf',fld,' Valve}'],'TexMode','on','horizontalAlignment', 'center')
      | text(0.5,0.08,['{----(P)}'],'TexMode','on','horizontalAlignment', 'center')
      | 
      | h      = get_param(gcb,'handle');   % Get block handle
      | blk    = gcb;
      | hblock = get(h);     % Parse out handles structure
      | for i = 1:str2num(hblock.Num_In)
      |     port_label('input',i,horzcat('Flow In #',num2str(i)))
      | end
      | port_label('input',4,'Input [u1 u2 u3]')
      | for i = 1:str2num(hblock.Num_Out)
      |     port_label('output',i,'Flow Out')
      | end

== system APST_Lib/Air Vehicle Components/Aircraft ==
  In1 : Inport
  Aircraft : MATLAB Function  TreatAsAtomicUnit=on
  Bus Creator2 : BusCreator  Inputs=1
  Data_Sink1 : APST_Lib/Support Components/Data_Sink
  Integrate : Integrator  InitialCondition=Vel_init
  Source1 : APST_Lib/Support Components/Source
  Source2 : APST_Lib/Support Components/Source
  b1 : BusCreator  Inputs=2
  b2 : BusCreator  Inputs=2
  Out1 : Outport
  Out2 : Outport  Port=2
  wires:
  Source2/1 -> [Thrust_2]
  Source1/1 -> [Thrust_1]
  [Thrust_2] -> b2/2  "Thrust"
  [Vel] -> b2/1  "Velocity"
  b2/1 -> Out2/1
  [Thrust_1] -> b1/2  "Thrust"
  [Vel] -> b1/1  "Velocity"
  b1/1 -> Out1/1
  [Thrust_1] -> Aircraft/2(Thrust_1)
  [Thrust_2] -> Aircraft/3(Thrust_2)
  Aircraft/1(x_dot) -> Integrate/1
  Integrate/1 -> [Vel], Aircraft/1(x)
  [M_fuel] -> Aircraft/4(M_fuel)
  Bus Creator2/1 -> Data_Sink1/1
  [Vel] -> Bus Creator2/1  "Velocity"
  In1/1 -> [M_fuel]

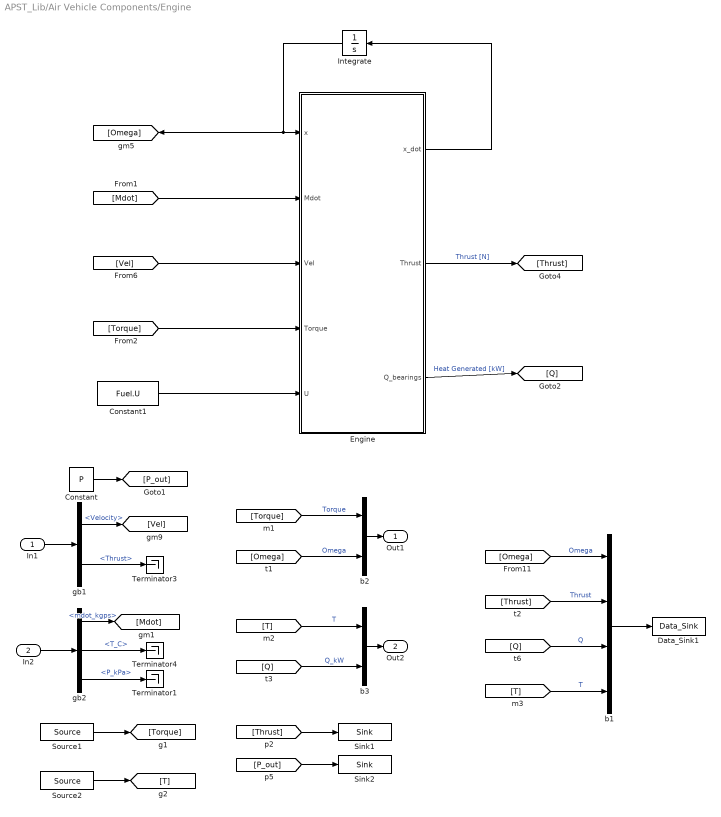
== system APST_Lib/Air Vehicle Components/Engine ==
  In1 : Inport
  In2 : Inport  Port=2
  Constant : Constant  Value=P
  Constant1 : Constant  Value=Fuel.U
  Data_Sink1 : APST_Lib/Support Components/Data_Sink
  Engine : MATLAB Function  TreatAsAtomicUnit=on
  Integrate : Integrator  InitialCondition=[Omega_init]
  Sink1 : APST_Lib/Support Components/Sink
  Sink2 : APST_Lib/Support Components/Sink
  Source1 : APST_Lib/Support Components/Source
  Source2 : APST_Lib/Support Components/Source
  Terminator1 : Terminator
  Terminator3 : Terminator
  Terminator4 : Terminator
  b1 : BusCreator  Inputs=4
  b2 : BusCreator  Inputs=2
  b3 : BusCreator  Inputs=2
  gb1 : BusSelector  OutputSignals=Velocity,Thrust
  gb2 : BusSelector  OutputSignals=mdot_kgps,T_C,P_kPa
  Out1 : Outport
  Out2 : Outport  Port=2
  wires:
  gb2/2 -> Terminator4/1  "<T_C>"
  gb2/1 -> [Mdot]  "<mdot_kgps>"
  In2/1 -> gb2/1
  gb2/3 -> Terminator1/1  "<P_kPa>"
  [P_out] -> Sink2/1
  b1/1 -> Data_Sink1/1
  [Omega] -> b1/1  "Omega"
  Constant/1 -> [P_out]
  Engine/1(x_dot) -> Integrate/1
  Engine/2(Thrust) -> [Thrust]  "Thrust [N]"
  Integrate/1 -> [Omega], Engine/1(x)
  [Mdot] -> Engine/2(Mdot)
  [Vel] -> Engine/3(Vel)
  [Torque] -> Engine/4(Torque)
  Constant1/1 -> Engine/5(U)
  [Thrust] -> b1/2  "Thrust"
  Engine/3(Q_bearings) -> [Q]  "Heat Generated [kW]"
  [Q] -> b1/3  "Q"
  b2/1 -> Out1/1
  [Torque] -> b2/1  "Torque"
  [Omega] -> b2/2  "Omega"
  Source1/1 -> [Torque]
  gb1/2 -> Terminator3/1  "<Thrust>"
  gb1/1 -> [Vel]  "<Velocity>"
  In1/1 -> gb1/1
  [Thrust] -> Sink1/1
  Source2/1 -> [T]
  b3/1 -> Out2/1
  [T] -> b3/1  "T"
  [Q] -> b3/2  "Q_kW"
  [T] -> b1/4  "T"

== system APST_Lib/Electrical Components/Battery ==
  In1 : Inport
  In2 : Inport  Port=2
  Battery : MATLAB Function  TreatAsAtomicUnit=on
  Bus Selector : BusSelector  OutputSignals=V,I
  Data_Sink1 : APST_Lib/Support Components/Data_Sink
  Integrate : Integrator  InitialCondition=[SOC0]
  P : Constant  Value=P_max
  Product : Product
  Sink1 : APST_Lib/Support Components/Sink
  Source1 : APST_Lib/Support Components/Source
  Terminator3 : Terminator
  b1 : BusCreator  Inputs=3
  b2 : BusCreator  Inputs=2
  eta : Fcn  Expr=a*u^2+b*u+c
  Out1 : Outport
  wires:
  Bus Selector/1 -> [V_in]  "<V>"
  Bus Selector/2 -> Terminator3/1  "<I>"
  [I_in] -> Sink1/1  "I"
  In1/1 -> Bus Selector/1
  P/1 -> Product/1
  In2/1 -> Product/2
  b1/1 -> Data_Sink1/1
  [P] -> b1/2  "Power"
  b2/1 -> Out1/1
  [T] -> b2/1  "T"
  [Q] -> b2/2  "Q_kW"
  Source1/1 -> [T]
  Battery/3(Q) -> [Q]
  Product/1 -> [P]  "Power"
  [Q] -> b1/3  "Q_kW"
  [SOC] -> b1/1  "SOC"
  [T] -> eta/1
  eta/1 -> [eta]
  Battery/1(x_dot) -> Integrate/1
  Integrate/1 -> Battery/1(x), [SOC]
  [eta] -> Battery/4(eta)
  [P] -> Battery/3(P)
  [V_in] -> Battery/2(V_in)
  Battery/2(I_in) -> [I_in]

== system APST_Lib/Electrical Components/Bus1 ==
  In : Inport
  Add : Sum
  Bus Creator1 : BusCreator  Inputs=2
  Bus Creator2 : BusCreator  Inputs=2
  Bus Selector : BusSelector  OutputSignals=V,I
  Sink1 : APST_Lib/Support Components/Sink
  Source1 : APST_Lib/Support Components/Source
  Source2 : APST_Lib/Support Components/Source
  Terminator3 : Terminator
  Out1 : Outport
  Out2 : Outport  Port=2
  wires:
  Source1/1 -> Add/1, Bus Creator1/2  "I"
  Bus Selector/2 -> Terminator3/1  "<I>"
  In/1 -> Bus Selector/1
  Bus Creator1/1 -> Out1/1
  Bus Selector/1 -> Bus Creator2/1, Bus Creator1/1  "<V>"
  Bus Creator2/1 -> Out2/1
  Source2/1 -> Add/2, Bus Creator2/2  "I"
  Add/1 -> Sink1/1

== system APST_Lib/Electrical Components/Converter ==
  In1 : Inport
  Constant : Constant  Value=V
  Constant1 : Constant  Value=0
  Converter : MATLAB Function  TreatAsAtomicUnit=on
  Data_Sink1 : APST_Lib/Support Components/Data_Sink
  Sink1 : APST_Lib/Support Components/Sink
  Source1 : APST_Lib/Support Components/Source
  Source2 : APST_Lib/Support Components/Source
  Switch : Switch  Criteria=u2 > Threshold
  Terminator2 : Terminator
  b1 : BusCreator  Inputs=5
  b2 : BusCreator  Inputs=2
  b3 : BusCreator  Inputs=2
  gb1 : BusSelector  OutputSignals=V,I
  Out1 : Outport
  Out2 : Outport  Port=2
  wires:
  [I_in] -> Sink1/1
  b1/1 -> Data_Sink1/1
  gb1/1 -> [V_in]  "<V>"
  In1/1 -> gb1/1
  gb1/2 -> Terminator2/1  "<I>"
  Converter/1(I_in) -> [I_in]  "I"
  [I_in] -> b1/1  "Current_in"
  Converter/2(Q) -> [Q]  "Heat Generated [kW]"
  [Q] -> b1/3  "Q_kW"
  b2/1 -> Out1/1
  [V] -> b2/1  "V"
  [I] -> b2/2  "I"
  [I] -> Converter/2(I)
  [V_in] -> Converter/1(V_in)
  Source1/1 -> [I]
  [I] -> b1/2  "Current"
  Constant1/1 -> Switch/3
  Constant/1 -> Switch/1
  Switch/1 -> [V]
  [V_in] -> Switch/2
  Converter/3(eta) -> [eta]  "eta"
  [eta] -> b1/4  "eta"
  Source2/1 -> [T]
  b3/1 -> Out2/1
  [T] -> b3/1  "T"
  [Q] -> b3/2  "Q_kW"
  [T] -> b1/5  "T"

== system APST_Lib/Electrical Components/Dist ==
  In1 : Inport
  In2 : Inport  Port=2
  u : Inport  Port=3
  Bus Creator1 : BusCreator  Inputs=2
  Bus Selector : BusSelector  OutputSignals=V,I
  Bus Selector1 : BusSelector  OutputSignals=V,I
  Constant : Constant  Value=0
  Demux : Demux  Outputs=2
  MinMax : MinMax
  Mux : Mux  Inputs=2
  Product : Product  Multiplication=Matrix(*)
  Sink1 : APST_Lib/Support Components/Sink
  Sink2 : APST_Lib/Support Components/Sink
  Source1 : APST_Lib/Support Components/Source
  Switch : Switch  Criteria=u2 > Threshold
  Terminator1 : Terminator
  Terminator3 : Terminator
  Out : Outport
  wires:
  [I] -> Bus Creator1/2  "I"
  Bus Selector/2 -> Terminator3/1  "<I>"
  In1/1 -> Bus Selector/1
  Bus Creator1/1 -> Out/1
  Bus Selector/1 -> Mux/1  "<V>"
  Source1/1 -> [I]  "I"
  Bus Selector1/2 -> Terminator1/1  "<I>"
  In2/1 -> Bus Selector1/1
  Bus Selector1/1 -> Mux/2  "<V>"
  MinMax/1 -> Switch/2, [V]  "Voltage"
  Switch/1 -> [I_ins]  "Current"
  [I] -> Product/2
  [V_ins] -> MinMax/1
  Mux/1 -> [V_ins]
  u/1 -> [u]
  [V] -> Bus Creator1/1  "V"
  [I_ins] -> Demux/1
  Demux/2 -> Sink2/1
  Demux/1 -> Sink1/1
  [u] -> Product/1
  Constant/1 -> Switch/3
  Product/1 -> Switch/1  "Current"

== system APST_Lib/Electrical Components/Generator ==
  In1 : Inport
  Constant : Constant  Value=V
  Data_Sink1 : APST_Lib/Support Components/Data_Sink
  Generator : MATLAB Function  TreatAsAtomicUnit=on
  Sink1 : APST_Lib/Support Components/Sink
  Source1 : APST_Lib/Support Components/Source
  Source2 : APST_Lib/Support Components/Source
  Terminator2 : Terminator
  b1 : BusCreator  Inputs=4
  b2 : BusCreator  Inputs=2
  b3 : BusCreator  Inputs=2
  gb1 : BusSelector  OutputSignals=Torque,Omega
  Out1 : Outport
  Out2 : Outport  Port=2
  wires:
  [Torque] -> Sink1/1
  b1/1 -> Data_Sink1/1
  gb1/1 -> Terminator2/1  "<Torque>"
  In1/1 -> gb1/1
  gb1/2 -> [Omega]  "<Omega>"
  Constant/1 -> [V]
  Generator/1(Torque) -> [Torque]  "Torque [Nm]"
  [Torque] -> b1/1  "Torque"
  Generator/2(Q) -> [Q]  "Heat Generated [kW]"
  [Q] -> b1/3  "Q_kW"
  b2/1 -> Out1/1
  [V] -> b2/1  "V"
  [I] -> b2/2  "I"
  [I] -> Generator/2(I)
  [Omega] -> Generator/1(Omega)
  Source1/1 -> [I]
  [I] -> b1/2  "Current"
  Source2/1 -> [T]
  b3/1 -> Out2/1
  [T] -> b3/1  "T"
  [Q] -> b3/2  "Q_kW"
  [T] -> b1/4  "T"

== system APST_Lib/Electrical Components/Heater ==
  In1 : Inport
  In2 : Inport  Port=2
  Bus Selector : BusSelector  OutputSignals=V,I
  Constant : Constant  Value=0
  Constant1 : Constant  Value=0
  Data_Sink1 : APST_Lib/Support Components/Data_Sink
  Divide : Product  Inputs=/
  Gain : Gain  Gain=1000
  P : Constant  Value=P_max
  Product : Product
  Product1 : Product
  Sink1 : APST_Lib/Support Components/Sink
  Source1 : APST_Lib/Support Components/Source
  Switch : Switch  Criteria=u2 > Threshold
  Switch1 : Switch  Criteria=u2 > Threshold
  Terminator3 : Terminator
  b1 : BusCreator  Inputs=2
  b2 : BusCreator  Inputs=2
  Out1 : Outport
  wires:
  Bus Selector/1 -> Divide/1, Switch/2, Switch1/2  "<V>"
  Bus Selector/2 -> Terminator3/1  "<I>"
  Product1/1 -> Gain/1  "I"
  In1/1 -> Bus Selector/1
  P/1 -> Product/1
  In2/1 -> Product/2
  Switch/1 -> Product1/1
  Divide/1 -> Switch/1
  Constant/1 -> Switch/3
  b1/1 -> Data_Sink1/1
  Switch1/1 -> b1/1, Product1/2, [Q]  "Power"
  b2/1 -> Out1/1
  [T] -> b2/1  "T"
  [Q] -> b2/2  "Q_kW"
  Source1/1 -> [T]
  Constant1/1 -> Switch1/3
  Product/1 -> Switch1/1  "Power"
  [Q] -> b1/2  "Q_kW"
  Gain/1 -> Sink1/1
